simulink model "glycosis_sim"  (R2023a)
settings: Solver=ode1  StartTime=0.0  StopTime=600  FixedStep=0.001  RelTol=1e-3
values from neighbouring files (symbols this model uses):
  a = 0    [simulate_hover.m]
  b = 3.9351*10^(-6)    (= 3.9351e-06)    [simulate_hover.m]
undefined symbols (not defined in the file or in its folder): o_glycosis
libraries: dspsrcs4 x1
settings Model: Creator=kille  LastModifiedBy=Jacob
settings DataIOCC: ReturnWorkspaceOutputs=off

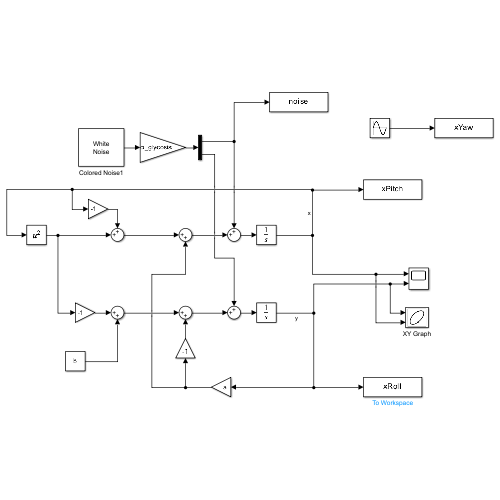
[thumbnail: Simulink's stored preview of the top-level diagram]
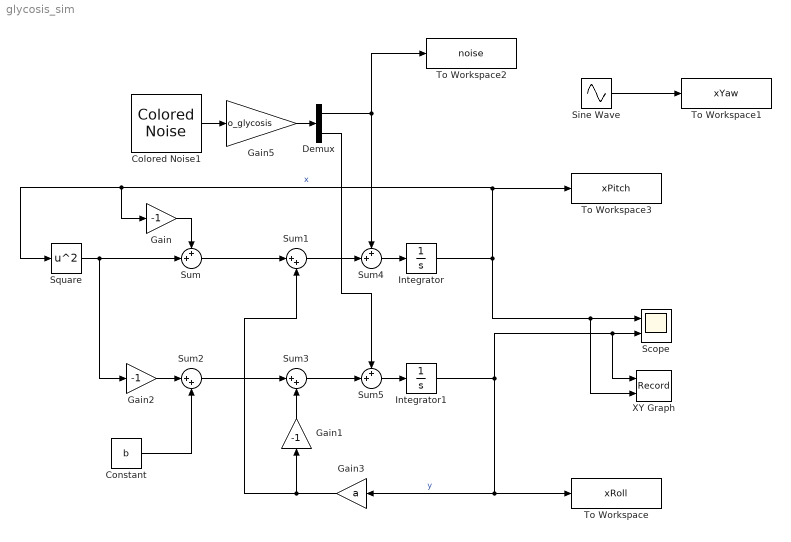
== system glycosis_sim ==
  Colored Noise1 : dspsrcs4/Colored Noise  Color=white  InverseFrequencyPower=1  BoundedOutput=off  NumChannels=2  OutputDataType=double  SamplesPerFrame=1  SampleTime=1  RandomStream=mt19937ar with seed  Seed=67  SimulateUsing=Interpreted execution
  Constant : Constant  Value=b
  Demux : Demux  Outputs=2
  Gain : Gain  Gain=-1
  Gain1 : Gain  Gain=-1
  Gain2 : Gain  Gain=-1
  Gain3 : Gain  Gain=a
  Gain5 : Gain  Gain=o_glycosis
  Integrator : Integrator
  Integrator1 : Integrator
  Scope : Scope  NumInputPorts=2
  Sine Wave : Sin  SampleTime=0
  Square : Math  Operator=square
  Sum : Sum  Inputs=++|
  Sum1 : Sum  Inputs=|++
  Sum2 : Sum  Inputs=|++
  Sum3 : Sum  Inputs=|++
  Sum4 : Sum  Inputs=++|
  Sum5 : Sum  Inputs=++|
  To Workspace : ToWorkspace  VariableName=xRoll  SampleTime=-1
  To Workspace1 : ToWorkspace  VariableName=xYaw  SampleTime=-1
  To Workspace2 : ToWorkspace  VariableName=noise  SaveFormat=Timeseries  SampleTime=-1
  To Workspace3 : ToWorkspace  VariableName=xPitch  SampleTime=-1
  XY Graph : Record  FileSettingsInternal="{\"entries\":[{\"content\":{\"excelSettings\":{\"content\":{},\"type\":\"Streamout.ExcelSettings\"}},\"type\":\"Streamout.FileSettingStorage\",\"uuid\":\"\"}],\"packageUris\":[\"http:\\/\\/schema.mathworks.com\\/mf0\\/streamout_blocks\\/R2020a\"],\"version\":\"1.0\"}"  Layout=[1 1]  SignalsInternal="{\"entries\":[{\"content\":{\"signals\":[{\"content\":{\"blockPath\":[],\"dimensions\":[1],\"domain\":\"\",\"lineColor\":\"#a2142f\",\"plots\":[1],\"port\":1,\"sid\":[\"\"],\"signalID\":1994,\"signalName\":\"y\"},\"type\":\"RecordBlkView.Signal\",\"uuid\":\"\"},{\"content\":{\"blockPath\":[],\"dimensions\":[1],\"domain\":\"\",\"lineColor\":\"#139fff\",\"plots\":[1],\"port\":2,\"sid\":[\"\"],\"signalID\":1998,\"signalName\":\"x\"},\"type\":\"RecordBlkView.Signal\",\"uuid\":\"\"}]},\"type\":\"RecordBlkView.InputSignals\",\"uuid\":\"\"}],\"packageUris\":[\"http:\\/\\/schema.mathworks.com\\/mf0\\/streamout_blocks\\/R2020a\"],\"version\":\"1.0\"}"  VisualizationBindings="{\"xyplotplugin\":{\"info\":[{\"series\":[{\"bindingParametersList\":[{\"parameter\":\"X-Axis\",\"signalID\":1994,\"signalName\":\"y\"},{\"parameter\":\"Y-Axis\",\"signalID\":1998,\"signalName\":\"x\"}],\"seriesID\":38349}],\"subplotID\":1}]}}"  CompatibilityTag=XY
  wires:
  Integrator/1 -> Square/1, Gain/1, To Workspace3/1, XY Graph/2, Scope/1  "x"
  Integrator1/1 -> To Workspace/1, Gain3/1, XY Graph/1, Scope/2  "y"
  Sum/1 -> Sum1/1
  Sum2/1 -> Sum3/1
  Square/1 -> Sum/2, Gain2/1
  Gain3/1 -> Gain1/1, Sum1/2
  Gain2/1 -> Sum2/1
  Gain/1 -> Sum/1
  Constant/1 -> Sum2/2
  Gain1/1 -> Sum3/2
  Colored Noise1/1 -> Gain5/1
  Sum5/1 -> Integrator1/1
  Sum3/1 -> Sum5/2
  Sum4/1 -> Integrator/1
  Sum1/1 -> Sum4/2
  Gain5/1 -> Demux/1
  Demux/1 -> To Workspace2/1, Sum4/1
  Demux/2 -> Sum5/1
  Sine Wave/1 -> To Workspace1/1
